simulink model "lab4"  (R2026a)
settings: Solver=VariableStepAuto  StopTime=24
settings Model: Creator=13676840  LastModifiedBy=gabriel

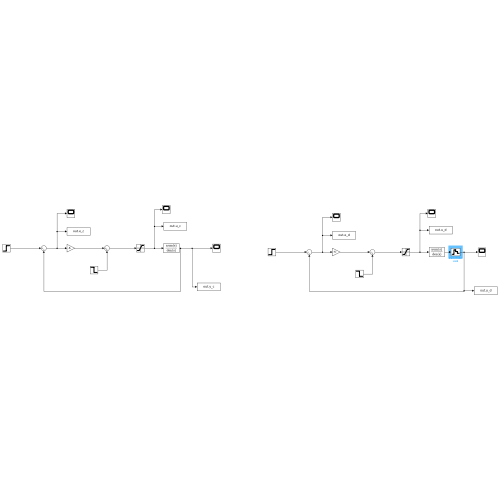
[thumbnail: Simulink's stored preview of the top-level diagram]
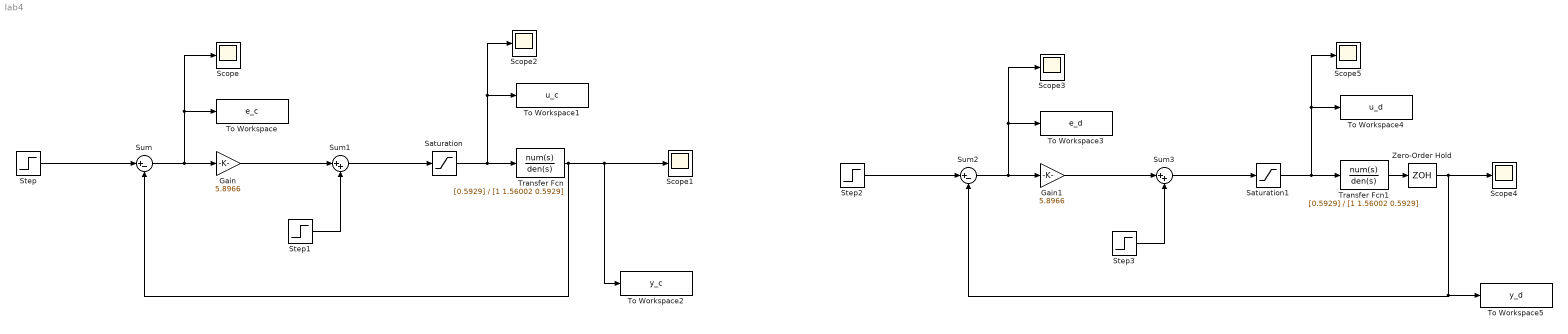
== system lab4 ==
  Gain : Gain  Gain=5.8966
  Gain1 : Gain  Gain=5.8966
  Saturation : Saturate  UpperLimit=10  LowerLimit=-10
  Saturation1 : Saturate  UpperLimit=10  LowerLimit=-10
  Scope{,1..5} (6 alike) : Scope
      Scope settings: ActiveDisplayYMinimum=0.48571  ActiveDisplayYMaximum=1.24603
      Scope2 settings: DataLoggingVariableName=ScopeData2
      Scope3 settings: ActiveDisplayYMinimum=0.48571  ActiveDisplayYMaximum=1.24603  DataLoggingVariableName=ScopeData3
      Scope4 settings: DataLoggingVariableName=ScopeData4
      Scope5 settings: DataLoggingVariableName=ScopeData5
  Step : Step  Time=0  FinalValue=1.17  SampleTime=0
  Step1 : Step  Time=12  FinalValue=-0.15  SampleTime=0
  Step2 : Step  Time=0  FinalValue=1.17  SampleTime=0
  Step3 : Step  Time=12  FinalValue=-0.15  SampleTime=0
  Sum : Sum  Inputs=|+-
  Sum1 : Sum  Inputs=|++
  Sum2 : Sum  Inputs=|+-
  Sum3 : Sum  Inputs=|++
  To Workspace : ToWorkspace  VariableName=e_c  SaveFormat=Timeseries  SampleTime=-1
  To Workspace1 : ToWorkspace  VariableName=u_c  SaveFormat=Timeseries  SampleTime=-1
  To Workspace2 : ToWorkspace  VariableName=y_c  SaveFormat=Timeseries  SampleTime=-1
  To Workspace3 : ToWorkspace  VariableName=e_d  SaveFormat=Timeseries  SampleTime=-1
  To Workspace4 : ToWorkspace  VariableName=u_d  SaveFormat=Timeseries  SampleTime=-1
  To Workspace5 : ToWorkspace  VariableName=y_d  SaveFormat=Timeseries  SampleTime=-1
  Transfer Fcn : TransferFcn  Numerator=[0.5929]  Denominator=[1 1.56002 0.5929]
  Transfer Fcn1 : TransferFcn  Numerator=[0.5929]  Denominator=[1 1.56002 0.5929]
  Zero-Order Hold : ZeroOrderHold  SampleTime=0.0897
  wires:
  Step/1 -> Sum/1
  Gain/1 -> Sum1/1
  Sum1/1 -> Saturation/1
  Saturation/1 -> To Workspace1/1, Scope2/1, Transfer Fcn/1
  Transfer Fcn/1 -> Sum/2, To Workspace2/1, Scope1/1
  Step1/1 -> Sum1/2
  Sum/1 -> To Workspace/1, Scope/1, Gain/1
  Step3/1 -> Sum3/2
  Sum2/1 -> To Workspace3/1, Scope3/1, Gain1/1
  Gain1/1 -> Sum3/1
  Sum3/1 -> Saturation1/1
  Saturation1/1 -> To Workspace4/1, Scope5/1, Transfer Fcn1/1
  Step2/1 -> Sum2/1
  Transfer Fcn1/1 -> Zero-Order Hold/1
  Zero-Order Hold/1 -> To Workspace5/1, Sum2/2, Scope4/1
